simulink model "collision_between_two_robots"  (R2018a)
settings: Solver=VariableStepAuto  StartTime=0.0  StopTime=120  FixedStep=0.01  MaxStep=.01  RelTol=1e-3
settings Model: Creator=U500304  LastModifiedBy=U500304
settings SolverCC: ZeroCrossAlgorithm=Adaptive
settings DataIOCC: SaveOutput=off  SaveTime=off
settings DebuggingCC: MaxConsecutiveZCsMsg=warning

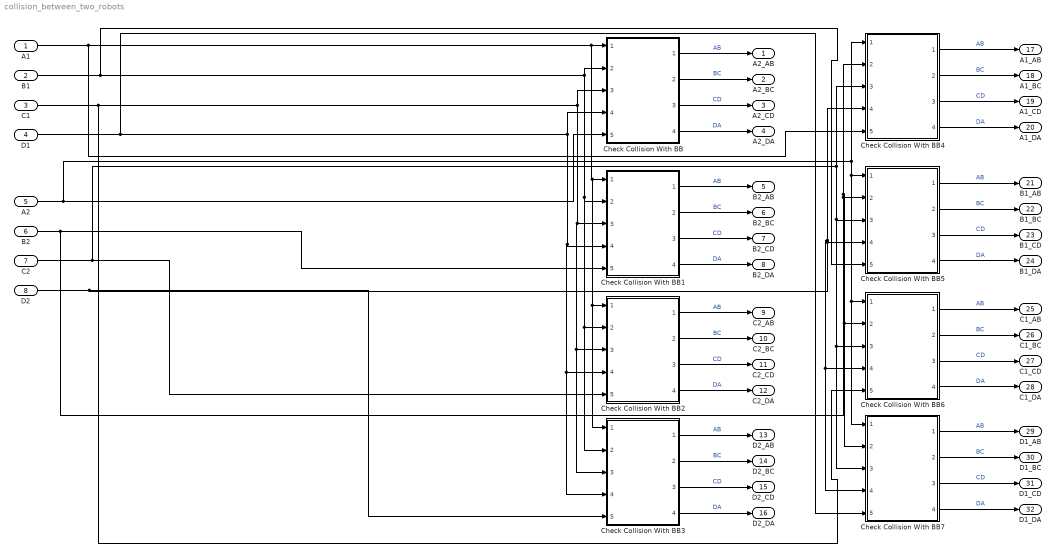
== system collision_between_two_robots ==
  A1 : Inport  OutDataTypeStr=double  PortDimensions=2
  B1 : Inport  Port=2  OutDataTypeStr=double  PortDimensions=2
  C1 : Inport  Port=3  OutDataTypeStr=double  PortDimensions=2
  D1 : Inport  Port=4  OutDataTypeStr=double  PortDimensions=2
  A2 : Inport  Port=5  OutDataTypeStr=double  PortDimensions=2
  B2 : Inport  Port=6  OutDataTypeStr=double  PortDimensions=2
  C2 : Inport  Port=7  OutDataTypeStr=double  PortDimensions=2
  D2 : Inport  Port=8  OutDataTypeStr=double  PortDimensions=2
  Check Collision With BB{,1..7} (8 alike) : ModelReference  ModelNameDialog=check_collision_with_bounding  SimulationMode=Normal  ModelReferenceVersion=1.644
  A2_AB : Outport  OutDataTypeStr=double  PortDimensions=1  SampleTime=0
  A2_BC : Outport  Port=2  OutDataTypeStr=double  PortDimensions=1  SampleTime=0
  A2_CD : Outport  Port=3  OutDataTypeStr=double  PortDimensions=1  SampleTime=0
  A2_DA : Outport  Port=4  OutDataTypeStr=double  PortDimensions=1  SampleTime=0
  B2_AB : Outport  Port=5  OutDataTypeStr=double  PortDimensions=1  SampleTime=0
  B2_BC : Outport  Port=6  OutDataTypeStr=double  PortDimensions=1  SampleTime=0
  B2_CD : Outport  Port=7  OutDataTypeStr=double  PortDimensions=1  SampleTime=0
  B2_DA : Outport  Port=8  OutDataTypeStr=double  PortDimensions=1  SampleTime=0
  C2_AB : Outport  Port=9  OutDataTypeStr=double  PortDimensions=1  SampleTime=0
  C2_BC : Outport  Port=10  OutDataTypeStr=double  PortDimensions=1  SampleTime=0
  C2_CD : Outport  Port=11  OutDataTypeStr=double  PortDimensions=1  SampleTime=0
  C2_DA : Outport  Port=12  OutDataTypeStr=double  PortDimensions=1  SampleTime=0
  D2_AB : Outport  Port=13  OutDataTypeStr=double  PortDimensions=1  SampleTime=0
  D2_BC : Outport  Port=14  OutDataTypeStr=double  PortDimensions=1  SampleTime=0
  D2_CD : Outport  Port=15  OutDataTypeStr=double  PortDimensions=1  SampleTime=0
  D2_DA : Outport  Port=16  OutDataTypeStr=double  PortDimensions=1  SampleTime=0
  A1_AB : Outport  Port=17  OutDataTypeStr=double  PortDimensions=1  SampleTime=0
  A1_BC : Outport  Port=18  OutDataTypeStr=double  PortDimensions=1  SampleTime=0
  A1_CD : Outport  Port=19  OutDataTypeStr=double  PortDimensions=1  SampleTime=0
  A1_DA : Outport  Port=20  OutDataTypeStr=double  PortDimensions=1  SampleTime=0
  B1_AB : Outport  Port=21  OutDataTypeStr=double  PortDimensions=1  SampleTime=0
  B1_BC : Outport  Port=22  OutDataTypeStr=double  PortDimensions=1  SampleTime=0
  B1_CD : Outport  Port=23  OutDataTypeStr=double  PortDimensions=1  SampleTime=0
  B1_DA : Outport  Port=24  OutDataTypeStr=double  PortDimensions=1  SampleTime=0
  C1_AB : Outport  Port=25  OutDataTypeStr=double  PortDimensions=1  SampleTime=0
  C1_BC : Outport  Port=26  OutDataTypeStr=double  PortDimensions=1  SampleTime=0
  C1_CD : Outport  Port=27  OutDataTypeStr=double  PortDimensions=1  SampleTime=0
  C1_DA : Outport  Port=28  OutDataTypeStr=double  PortDimensions=1  SampleTime=0
  D1_AB : Outport  Port=29  OutDataTypeStr=double  PortDimensions=1  SampleTime=0
  D1_BC : Outport  Port=30  OutDataTypeStr=double  PortDimensions=1  SampleTime=0
  D1_CD : Outport  Port=31  OutDataTypeStr=double  PortDimensions=1  SampleTime=0
  D1_DA : Outport  Port=32  OutDataTypeStr=double  PortDimensions=1  SampleTime=0
  wires:
  Check Collision With BB3/3 -> D2_CD/1  "CD"
  Check Collision With BB2/3 -> C2_CD/1  "CD"
  Check Collision With BB/4 -> A2_DA/1  "DA"
  Check Collision With BB/3 -> A2_CD/1  "CD"
  Check Collision With BB1/3 -> B2_CD/1  "CD"
  Check Collision With BB1/2 -> B2_BC/1  "BC"
  Check Collision With BB2/1 -> C2_AB/1  "AB"
  Check Collision With BB1/4 -> B2_DA/1  "DA"
  Check Collision With BB/1 -> A2_AB/1  "AB"
  Check Collision With BB1/1 -> B2_AB/1  "AB"
  Check Collision With BB/2 -> A2_BC/1  "BC"
  Check Collision With BB2/2 -> C2_BC/1  "BC"
  Check Collision With BB3/4 -> D2_DA/1  "DA"
  Check Collision With BB2/4 -> C2_DA/1  "DA"
  Check Collision With BB3/1 -> D2_AB/1  "AB"
  Check Collision With BB3/2 -> D2_BC/1  "BC"
  Check Collision With BB6/3 -> C1_CD/1  "CD"
  Check Collision With BB7/3 -> D1_CD/1  "CD"
  Check Collision With BB7/1 -> D1_AB/1  "AB"
  Check Collision With BB6/1 -> C1_AB/1  "AB"
  Check Collision With BB7/4 -> D1_DA/1  "DA"
  Check Collision With BB7/2 -> D1_BC/1  "BC"
  Check Collision With BB4/4 -> A1_DA/1  "DA"
  Check Collision With BB5/1 -> B1_AB/1  "AB"
  Check Collision With BB5/4 -> B1_DA/1  "DA"
  Check Collision With BB5/2 -> B1_BC/1  "BC"
  Check Collision With BB4/3 -> A1_CD/1  "CD"
  Check Collision With BB5/3 -> B1_CD/1  "CD"
  D2/1 -> Check Collision With BB3/5, Check Collision With BB5/4, Check Collision With BB6/4, Check Collision With BB7/4, Check Collision With BB4/4
  Check Collision With BB4/1 -> A1_AB/1  "AB"
  B2/1 -> Check Collision With BB1/5, Check Collision With BB5/2, Check Collision With BB6/2, Check Collision With BB7/2, Check Collision With BB4/2
  B1/1 -> Check Collision With BB1/2, Check Collision With BB2/2, Check Collision With BB3/2, Check Collision With BB/2, Check Collision With BB5/5
  C1/1 -> Check Collision With BB1/3, Check Collision With BB2/3, Check Collision With BB3/3, Check Collision With BB/3, Check Collision With BB6/5
  D1/1 -> Check Collision With BB1/4, Check Collision With BB2/4, Check Collision With BB3/4, Check Collision With BB/4, Check Collision With BB7/5
  C2/1 -> Check Collision With BB2/5, Check Collision With BB5/3, Check Collision With BB6/3, Check Collision With BB7/3, Check Collision With BB4/3
  Check Collision With BB6/2 -> C1_BC/1  "BC"
  A2/1 -> Check Collision With BB/5, Check Collision With BB5/1, Check Collision With BB6/1, Check Collision With BB7/1, Check Collision With BB4/1
  Check Collision With BB4/2 -> A1_BC/1  "BC"
  A1/1 -> Check Collision With BB1/1, Check Collision With BB2/1, Check Collision With BB3/1, Check Collision With BB/1, Check Collision With BB4/5
  Check Collision With BB6/4 -> C1_DA/1  "DA"
